simulink subsystem "Automotive_Suspension_Tire2Veh"  (R2024a)
settings: Solver=VariableStepAuto  StartTime=0.0  StopTime=10.0  RelTol=1e-3
libraries: sharedtransform x2
settings Model: Creator=USER  LastModifiedBy=USER

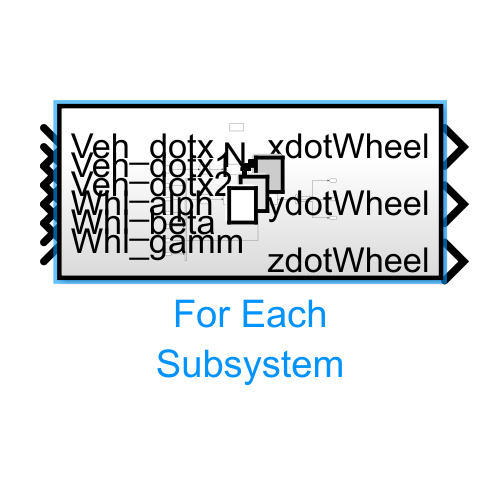
[thumbnail: Simulink's stored preview of the top-level diagram]
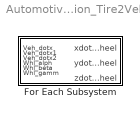
== system Automotive_Suspension_Tire2Veh ==
  For Each Subsystem : Subsystem  TreatAsAtomicUnit=on

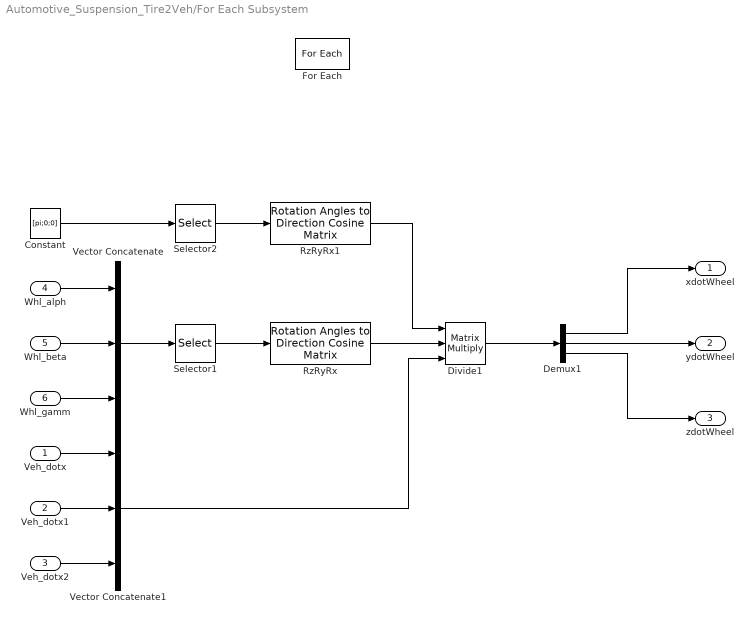
== system Automotive_Suspension_Tire2Veh/For Each Subsystem ==
  Veh_dotx : Inport  Partition=on  PartitionDimension=1  PartitionWidth=1  PartitionOffset=0
  Veh_dotx1 : Inport  Port=2  Partition=on  PartitionDimension=1  PartitionWidth=1  PartitionOffset=0
  Veh_dotx2 : Inport  Port=3  Partition=on  PartitionDimension=1  PartitionWidth=1  PartitionOffset=0
  Whl_alph : Inport  Port=4  Partition=on  PartitionDimension=1  PartitionWidth=1  PartitionOffset=0
  Whl_beta : Inport  Port=5  Partition=on  PartitionDimension=1  PartitionWidth=1  PartitionOffset=0
  Whl_gamm : Inport  Port=6  Partition=on  PartitionDimension=1  PartitionWidth=1  PartitionOffset=0
  Constant : Constant  Value=[pi;0;0]
  Demux1 : Demux  Outputs=3
  Divide1 : Product  Inputs=***  Multiplication=Matrix(*)
  For Each : ForEach  DisableCoverage=on
  RzRyRx : sharedtransform/Rotation Angles to Direction Cosine Matrix  rotationOrder=ZYX  aMode=aMode
  RzRyRx1 : sharedtransform/Rotation Angles to Direction Cosine Matrix  rotationOrder=ZYX  aMode=aMode
  Selector1 : Selector  InputPortWidth=3  IndexOptions=Index vector (dialog)  Indices=[3 2 1]  OutputSizes=1
  Selector2 : Selector  InputPortWidth=3  IndexOptions=Index vector (dialog)  Indices=[3 2 1]  OutputSizes=1
  Vector Concatenate : Concatenate  NumInputs=3
  Vector Concatenate1 : Concatenate  NumInputs=3
  xdotWheel : Outport  ConcatenationDimension=1  VectorParamsAs1DForOutWhenUnconnected=off
  ydotWheel : Outport  Port=2  ConcatenationDimension=1  VectorParamsAs1DForOutWhenUnconnected=off
  zdotWheel : Outport  Port=3  ConcatenationDimension=1  VectorParamsAs1DForOutWhenUnconnected=off
  wires:
  Whl_alph/1 -> Vector Concatenate/1
  Whl_beta/1 -> Vector Concatenate/2
  Whl_gamm/1 -> Vector Concatenate/3
  Vector Concatenate/1 -> Selector1/1
  Selector1/1 -> RzRyRx/1
  Constant/1 -> Selector2/1
  Selector2/1 -> RzRyRx1/1
  RzRyRx1/1 -> Divide1/1
  RzRyRx/1 -> Divide1/2
  Divide1/1 -> Demux1/1
  Demux1/1 -> xdotWheel/1
  Demux1/2 -> ydotWheel/1
  Demux1/3 -> zdotWheel/1
  Veh_dotx/1 -> Vector Concatenate1/1
  Veh_dotx1/1 -> Vector Concatenate1/2
  Veh_dotx2/1 -> Vector Concatenate1/3
  Vector Concatenate1/1 -> Divide1/3
